simulink library "MFMdl5"  (Simulink 8.8)
settings: Solver=VariableStepAuto  StartTime=0.0  StopTime=10.0  RelTol=1e-3
libraries: simulink x4
settings Model: Creator=viett  LastModifiedBy=viett

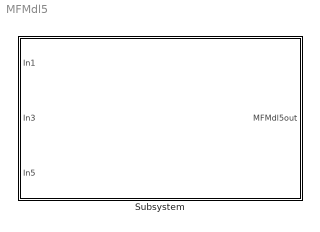
== system MFMdl5 ==
  Subsystem : Subsystem

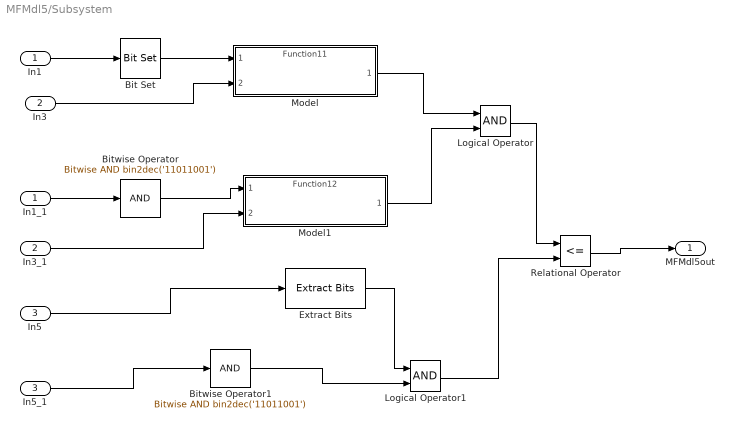
== system MFMdl5/Subsystem ==
  In1 : Inport
  In3 : Inport  Port=2
  In5 : Inport  Port=3
  Bit Set : simulink/Logic and Bit Operations/Bit Set  iBit=0
  Bitwise Operator : simulink/Logic and Bit Operations/Bitwise Operator  logicop=AND  UseBitMask=on  BitMask=bin2dec('11011001')  BitMaskRealWorld=Stored Integer
  Bitwise Operator1 : simulink/Logic and Bit Operations/Bitwise Operator  logicop=AND  UseBitMask=on  BitMask=bin2dec('11011001')  BitMaskRealWorld=Stored Integer
  Extract Bits : simulink/Logic and Bit Operations/Extract Bits  bitsToExtract=Upper half  numBits=8  bitIdxRange=[0 7]  outScalingMode=Preserve fixed-point scaling
  In1_1 : InportShadow
  In3_1 : InportShadow  Port=2
  In5_1 : InportShadow  Port=3
  Logical Operator : Logic  AllPortsSameDT=off  OutDataTypeStr=boolean
  Logical Operator1 : Logic  AllPortsSameDT=off  OutDataTypeStr=boolean
  Model : ModelReference  ModelNameDialog=Function11.slx  SimulationMode=Normal  ModelReferenceVersion=1.20
  Model1 : ModelReference  ModelNameDialog=Function12.slx  SimulationMode=Normal  ModelReferenceVersion=1.18
  Relational Operator : RelationalOperator  Operator=<=  OutDataTypeStr=boolean  RndMeth=Simplest
  MFMdl5out : Outport
  wires:
  In3_1/1 -> Model1/2
  Bitwise Operator1/1 -> Logical Operator1/2
  Model1/1 -> Logical Operator/2
  Bit Set/1 -> Model/1
  Extract Bits/1 -> Logical Operator1/1
  Logical Operator/1 -> Relational Operator/1
  Logical Operator1/1 -> Relational Operator/2
  Bitwise Operator/1 -> Model1/1
  Model/1 -> Logical Operator/1
  In3/1 -> Model/2
  Relational Operator/1 -> MFMdl5out/1
  In5_1/1 -> Bitwise Operator1/1
  In1_1/1 -> Bitwise Operator/1
  In5/1 -> Extract Bits/1
  In1/1 -> Bit Set/1
